simulink model "simulink_model_traverse"  (R2021b)
settings: Solver=ode45  StartTime=0.0  StopTime=20  RelTol=1e-3
model workspace (MAT data in the model file):
  real_gyro_traverse_system : object (value not decoded)
values from neighbouring files (symbols this model uses):
  fric_gear_motor_traverse = 0.021    [loading_project.m]
  fric_gear_turrent_gun_traverse = 1.272    [loading_project.m]
  ts3 = 10^-3    (= 0.001)    [loading_project.m]
libraries: simulink x3, dspsrcs4 x1
(part 2 of 2)

== system simulink_model_traverse/linear plant traverse4/Coulomb_Friction_Model1 ==
  Torque : Inport
  velocity : Inport  Port=2
  velocity state : Inport  Port=3
  Abs2 : Abs  ZeroCross=off
  Gain : Gain  Gain=1.1
  Gain1 : Gain
  Hit Crossing : HitCross  ZeroCross=off
  MinMax : MinMax  Inputs=2
  Product1 : Product  RndMeth=Zero
  Product2 : Product  RndMeth=Zero
  Sign1 : Signum  ZeroCross=off
  Sign2 : Signum  ZeroCross=off
  Slip_T_friction : Constant  Value=fric_gear_turrent_gun_traverse  SampleTime=0
  Stick_T_friction : Constant  Value=fric_gear_turrent_gun_traverse  SampleTime=0
  Sw6 : Switch  Threshold=0.5  ZeroCross=off  SaturateOnIntegerOverflow=on  InputSameDT=on
  Friction_Torque : Outport
  reset velocity : Outport  Port=2
  wires:
  Torque/1 -> Sign2/1, Abs2/1
  Sw6/1 -> Friction_Torque/1
  Hit Crossing/1 -> reset velocity/1, Sw6/2
  Abs2/1 -> MinMax/2
  MinMax/1 -> Product2/1
  Product2/1 -> Sw6/1
  Product1/1 -> Sw6/3
  velocity/1 -> Sign1/1
  Sign1/1 -> Product1/2
  Sign2/1 -> Product2/2
  velocity state/1 -> Hit Crossing/1
  Gain/1 -> MinMax/1
  Stick_T_friction/1 -> Gain/1
  Slip_T_friction/1 -> Gain1/1
  Gain1/1 -> Product1/1

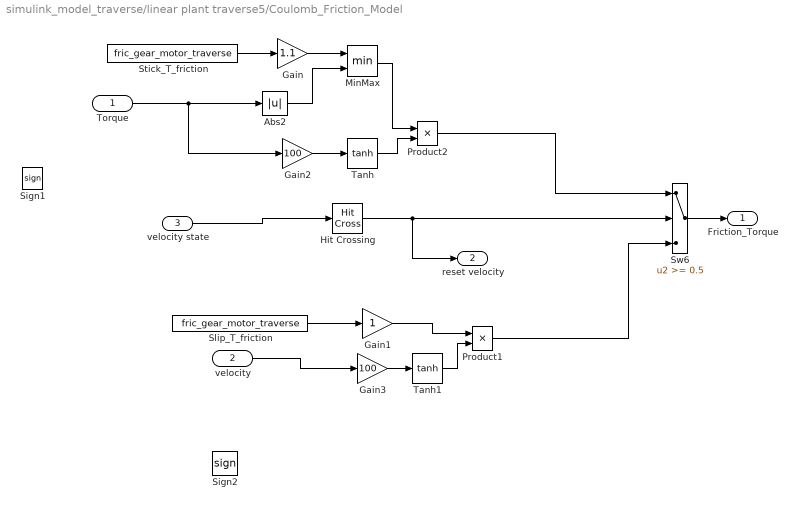
== system simulink_model_traverse/linear plant traverse5/Coulomb_Friction_Model ==
  Torque : Inport
  velocity : Inport  Port=2
  velocity state : Inport  Port=3
  Abs2 : Abs  ZeroCross=off
  Gain : Gain  Gain=1.1
  Gain1 : Gain
  Gain2 : Gain  Gain=100
  Gain3 : Gain  Gain=100
  Hit Crossing : HitCross  ZeroCross=off
  MinMax : MinMax  Inputs=2
  Product1 : Product  RndMeth=Zero
  Product2 : Product  RndMeth=Zero
  Sign1 : Signum  ZeroCross=off
  Sign2 : Signum  ZeroCross=off
  Slip_T_friction : Constant  Value=fric_gear_motor_traverse
  Stick_T_friction : Constant  Value=fric_gear_motor_traverse
  Sw6 : Switch  Threshold=0.5  ZeroCross=off  SaturateOnIntegerOverflow=on  InputSameDT=on
  Tanh : Trigonometry  Operator=tanh
  Tanh1 : Trigonometry  Operator=tanh
  Friction_Torque : Outport
  reset velocity : Outport  Port=2
  wires:
  Torque/1 -> Gain2/1, Abs2/1
  Sw6/1 -> Friction_Torque/1
  Hit Crossing/1 -> reset velocity/1, Sw6/2
  Abs2/1 -> MinMax/2
  MinMax/1 -> Product2/1
  Product2/1 -> Sw6/1
  Product1/1 -> Sw6/3
  velocity state/1 -> Hit Crossing/1
  Stick_T_friction/1 -> Gain/1
  Gain/1 -> MinMax/1
  Slip_T_friction/1 -> Gain1/1
  Gain1/1 -> Product1/1
  Gain2/1 -> Tanh/1
  Tanh/1 -> Product2/2
  velocity/1 -> Gain3/1
  Gain3/1 -> Tanh1/1
  Tanh1/1 -> Product1/2

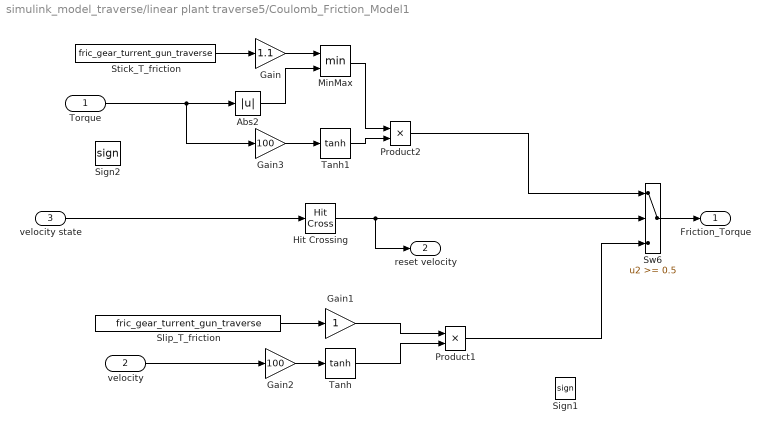
== system simulink_model_traverse/linear plant traverse5/Coulomb_Friction_Model1 ==
  Torque : Inport
  velocity : Inport  Port=2
  velocity state : Inport  Port=3
  Abs2 : Abs  ZeroCross=off
  Gain : Gain  Gain=1.1
  Gain1 : Gain
  Gain2 : Gain  Gain=100
  Gain3 : Gain  Gain=100
  Hit Crossing : HitCross  ZeroCross=off
  MinMax : MinMax  Inputs=2
  Product1 : Product  RndMeth=Zero
  Product2 : Product  RndMeth=Zero
  Sign1 : Signum  ZeroCross=off
  Sign2 : Signum  ZeroCross=off
  Slip_T_friction : Constant  Value=fric_gear_turrent_gun_traverse  SampleTime=0
  Stick_T_friction : Constant  Value=fric_gear_turrent_gun_traverse  SampleTime=0
  Sw6 : Switch  Threshold=0.5  ZeroCross=off  SaturateOnIntegerOverflow=on  InputSameDT=on
  Tanh : Trigonometry  Operator=tanh
  Tanh1 : Trigonometry  Operator=tanh
  Friction_Torque : Outport
  reset velocity : Outport  Port=2
  wires:
  Torque/1 -> Gain3/1, Abs2/1
  Sw6/1 -> Friction_Torque/1
  Hit Crossing/1 -> reset velocity/1, Sw6/2
  Abs2/1 -> MinMax/2
  MinMax/1 -> Product2/1
  Product2/1 -> Sw6/1
  Product1/1 -> Sw6/3
  velocity state/1 -> Hit Crossing/1
  Gain/1 -> MinMax/1
  Stick_T_friction/1 -> Gain/1
  Slip_T_friction/1 -> Gain1/1
  Gain1/1 -> Product1/1
  velocity/1 -> Gain2/1
  Gain2/1 -> Tanh/1
  Tanh/1 -> Product1/2
  Tanh1/1 -> Product2/2
  Gain3/1 -> Tanh1/1
